simulink model "ReceptionCodeManchester"  (Simulink 10.1)
settings: Solver=FixedStepDiscrete  StartTime=0.0  StopTime=1e4  FixedStep=0.1  RelTol=1e-3
libraries: simulink x2, commrandsrc3 x1, commfilt2 x1, commsink2 x1, dspsigops x1, commutil2 x1
settings Model: Creator=iba  LastModifiedBy=iba
settings DataIOCC: SaveFormat=Dataset  SaveOutput=off  SignalLogging=off  SaveTime=off  ReturnWorkspaceOutputs=on
settings OptimizationCC: DefaultParameterBehavior=Inlined  LifeSpan=auto
settings DebuggingCC: AlgebraicLoopMsg=error  UnderspecifiedInitializationDetection=Simplified  MergeDetectMultiDrivingBlocksExec=error  SingleTaskRateTransMsg=warning  SFUnexpectedBacktrackingDiag=error  SFNoUnconditionalDefaultTransitionDiag=error  SFExecutionAtInitializationDiag=warning  ArithmeticOperatorsInVariantConditions=error
settings HardwareCC: ProdBitPerPointer=64  ProdBitPerSizeT=64  ProdBitPerPtrDiffT=64  ProdLargestAtomicFloat=Float  ProdIntDivRoundTo=Zero  ProdEndianess=LittleEndian  ProdWordSize=64  ProdHWDeviceType=Intel->x86-64 (Windows64)
settings ModelReferenceCC: PropagateSignalLabelsOutOfModel=on
settings SFSimCC: SimUseLocalCustomCode=on  CustomCodeUndefinedFunction=FilterOut
settings RTWCC: RTWUseLocalCustomCode=on
settings CodeAppCC: StateflowObjectComments=off
settings GRTTargetCC: TargetLangStandard=C99 (ISO)  CombineOutputUpdateFcns=on  GRTInterface=off
settings ConfigComp: CovMetricSettings=dwe  CovHtmlReporting=off  CovSaveCumulativeToWorkspaceVar=off  CovSaveSingleToWorkspaceVar=off  CovExternalEMLEnable=on

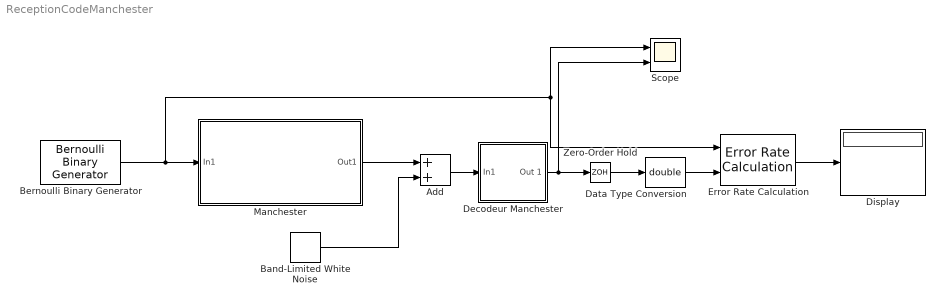
== system ReceptionCodeManchester ==
  Add : Sum
  Band-Limited White Noise : simulink/Sources/Band-Limited White Noise  Cov=1e-1  Ts=0.1  seed=[23341]
  Bernoulli Binary Generator : commrandsrc3/Bernoulli Binary Generator  ProbabilityOfZero=0.5  SeedSource=Parameter  Seed=61  SampleTime=1  SamplesPerFrame=1  OutputDataType=double  SimulateUsing=Interpreted execution
  Data Type Conversion : DataTypeConversion  OutDataTypeStr=double  LockScale=on
  Decodeur Manchester : Subsystem
  Display : Display
  Error Rate Calculation : commsink2/Error Rate Calculation  N=0  st_delay=0  cp_mode=Entire frame  subframe=[]  PMode=Port  WsName=ErrorVec  RsMode2=off  stop=off  numErr=100  maxBits=1e6
  Manchester : Subsystem
  Scope : Scope  NumInputPorts=2
  Zero-Order Hold : ZeroOrderHold
  wires:
  Band-Limited White Noise/1 -> Add/2
  Manchester/1(Out1) -> Add/1
  Bernoulli Binary Generator/1 -> Scope/1, Error Rate Calculation/1, Manchester/1("In1 ")
  Add/1 -> Decodeur Manchester/1("In1 ")
  Decodeur Manchester/1(Out 1) -> Scope/2, Zero-Order Hold/1
  Error Rate Calculation/1 -> Display/1
  Data Type Conversion/1 -> Error Rate Calculation/2
  Zero-Order Hold/1 -> Data Type Conversion/1

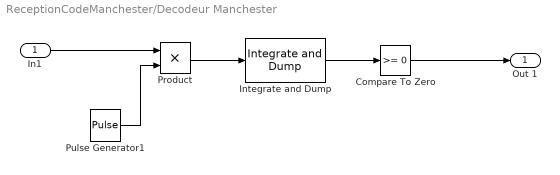
== system ReceptionCodeManchester/Decodeur Manchester ==
  "In1 " : Inport
  Compare To Zero : simulink/Logic and Bit Operations/Compare To Zero  relop=>=  OutDataTypeStr=boolean
  Integrate and Dump : commfilt2/Integrate and Dump  obssamples=10  offsetsamples=0  nodump=on  roundingMode=Floor  overflowMode=off  outputDataTypeStr=Inherit: Same as accumulator  outputLastDataTypeStr=Inherit: Same as accumulator
  Product : Product
  Pulse Generator1 : DiscretePulseGenerator  SampleTime=0.1
  Out 1 : Outport
  wires:
  Pulse Generator1/1 -> Product/2
  Product/1 -> Integrate and Dump/1
  Integrate and Dump/1 -> Compare To Zero/1
  Compare To Zero/1 -> Out 1/1
  "In1 "/1 -> Product/1

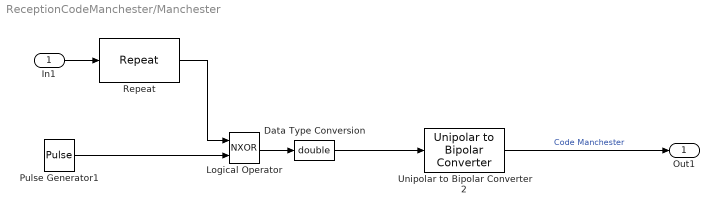
== system ReceptionCodeManchester/Manchester ==
  "In1 " : Inport
  "Data Type Conversion " : DataTypeConversion  OutDataTypeStr=double  LockScale=on
  Logical Operator : Logic  Operator=NXOR  AllPortsSameDT=off  OutDataTypeStr=boolean
  Pulse Generator1 : DiscretePulseGenerator  SampleTime=0.5
  Repeat : dspsigops/Repeat  N=2  InputProcessing=Columns as channels (frame based)  RateOptions=Allow multirate processing  ic=0  mode=Unused parameter value
  Unipolar to Bipolar Converter 2 : commutil2/Unipolar to Bipolar Converter  M=2  polarity=Positive  dataType=Inherit via internal rule
  Out1 : Outport
  wires:
  Pulse Generator1/1 -> Logical Operator/2
  Logical Operator/1 -> "Data Type Conversion "/1
  "In1 "/1 -> Repeat/1
  "Data Type Conversion "/1 -> Unipolar to Bipolar Converter 2/1
  Unipolar to Bipolar Converter 2/1 -> Out1/1  "Code Manchester"
  Repeat/1 -> Logical Operator/1
